simulink model "laser_cnc_openloop"  (R2024a)
settings: Solver=ode23t  StartTime=0.0  StopTime=0.5  RelTol=1e-3
settings Model: Creator=Sir Kiru  LastModifiedBy=Sir Kiru

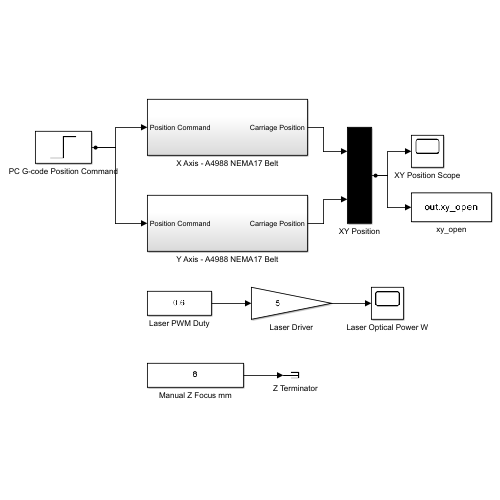
[thumbnail: Simulink's stored preview of the top-level diagram]
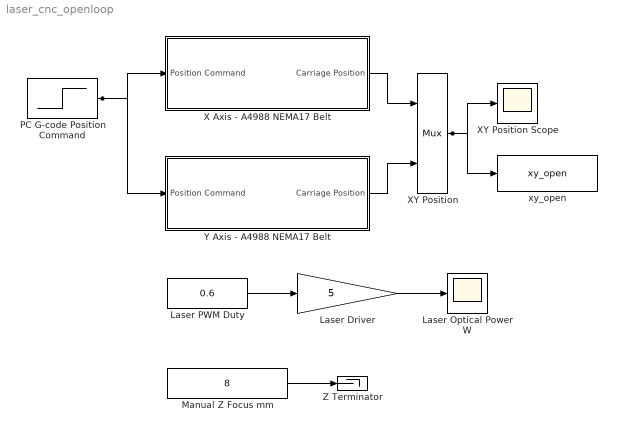
== system laser_cnc_openloop ==
  Laser Driver : Gain  Gain=5
  Laser Optical Power W : Scope
  Laser PWM Duty : Constant  Value=0.6
  Manual Z Focus mm : Constant  Value=8
  PC G-code Position Command : Step  Time=0.05  After=0.05  SampleTime=0
  X Axis - A4988 NEMA17 Belt : Subsystem
  XY Position : Mux  Inputs=2
  XY Position Scope : Scope
  Y Axis - A4988 NEMA17 Belt : Subsystem
  Z Terminator : Terminator
  xy_open : ToWorkspace  VariableName=xy_open  SaveFormat=Structure With Time  SampleTime=-1
  wires:
  PC G-code Position Command/1 -> X Axis - A4988 NEMA17 Belt/1(Position Command), Y Axis - A4988 NEMA17 Belt/1(Position Command)
  X Axis - A4988 NEMA17 Belt/1(Carriage Position) -> XY Position/1
  Y Axis - A4988 NEMA17 Belt/1(Carriage Position) -> XY Position/2
  XY Position/1 -> XY Position Scope/1, xy_open/1
  Laser PWM Duty/1 -> Laser Driver/1
  Laser Driver/1 -> Laser Optical Power W/1
  Manual Z Focus mm/1 -> Z Terminator/1

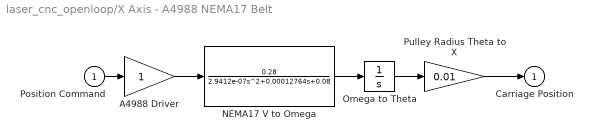
== system laser_cnc_openloop/X Axis - A4988 NEMA17 Belt ==
  Position Command : Inport
  A4988 Driver : Gain
  NEMA17 V to Omega : TransferFcn  Numerator=[0.28]  Denominator=[2.9412e-07 0.00012764 0.08]
  Omega to Theta : Integrator
  Pulley Radius Theta to X : Gain  Gain=0.01
  Carriage Position : Outport
  wires:
  Position Command/1 -> A4988 Driver/1
  A4988 Driver/1 -> NEMA17 V to Omega/1
  NEMA17 V to Omega/1 -> Omega to Theta/1
  Omega to Theta/1 -> Pulley Radius Theta to X/1
  Pulley Radius Theta to X/1 -> Carriage Position/1

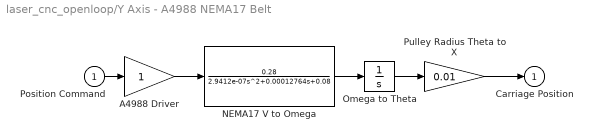
== system laser_cnc_openloop/Y Axis - A4988 NEMA17 Belt ==
  Position Command : Inport
  A4988 Driver : Gain
  NEMA17 V to Omega : TransferFcn  Numerator=[0.28]  Denominator=[2.9412e-07 0.00012764 0.08]
  Omega to Theta : Integrator
  Pulley Radius Theta to X : Gain  Gain=0.01
  Carriage Position : Outport
  wires:
  Position Command/1 -> A4988 Driver/1
  A4988 Driver/1 -> NEMA17 V to Omega/1
  NEMA17 V to Omega/1 -> Omega to Theta/1
  Omega to Theta/1 -> Pulley Radius Theta to X/1
  Pulley Radius Theta to X/1 -> Carriage Position/1
